simulink model "sunsensor_valid_flag_test"  (R2016b)
settings: Solver=VariableStepAuto  StartTime=0.0  StopTime=1  RelTol=1e-3
values from neighbouring files (symbols this model uses):
  alpha = -pi/6    (= -0.523598775598)    [sunsensor_valid_flag_test_init.m]
  beta = pi/2    (= 1.57079632679)    [sunsensor_valid_flag_test_init.m]
  fsw_params = init_fsw_params()    [sunsensor_processing_test_init.m]    (also in sunsensor_valid_flag_test_init.m)
  sun_vec_valid = 1    [sunsensor_valid_flag_test_init.m]
libraries: sensor_processing_libs x1
settings Model: Creator=sexymathemagician  LastModifiedBy=sexymathemagician

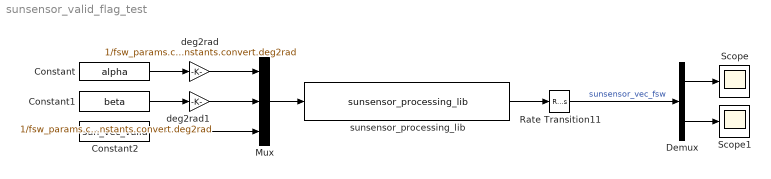
== system sunsensor_valid_flag_test ==
  Constant : Constant  Value=alpha
  Constant1 : Constant  Value=beta
  Constant2 : Constant  Value=sun_vec_valid
  Demux : Demux  Outputs=[3 1]
  Mux : Mux  Inputs=3
  Rate Transition11 : RateTransition  OutPortSampleTime=fsw_params.sample_time_s
  Scope : Scope
  Scope1 : Scope
  deg2rad : Gain  Gain=1/fsw_params.constants.convert.deg2rad
  deg2rad1 : Gain  Gain=1/fsw_params.constants.convert.deg2rad
  sunsensor_processing_lib : sensor_processing_libs/sunsensor_processing_lib
  wires:
  sunsensor_processing_lib/1 -> Rate Transition11/1
  Rate Transition11/1 -> Demux/1  "sunsensor_vec_fsw"
  Demux/1 -> Scope/1
  Demux/2 -> Scope1/1
  Mux/1 -> sunsensor_processing_lib/1
  Constant/1 -> deg2rad/1
  Constant1/1 -> deg2rad1/1
  Constant2/1 -> Mux/3
  deg2rad/1 -> Mux/1
  deg2rad1/1 -> Mux/2
